simulink model "uuvSim_mfsm"  (R2017b)
settings: Solver=ode4  StartTime=0.0  StopTime=10.0  FixedStep=mdl.tStep  RelTol=1e-3
values from neighbouring files (symbols this model uses):
  trj_type = block.DialogPrm(1).Data    [trj_gen.m]    (also in trj_gen_mpc.m)
  waypoints = block.DialogPrm(2).Data    [trj_gen.m]    (also in trj_gen_mpc.m)
undefined symbols (not defined in the file or in its folder): A, ics, Kd, Ki, mdl, rov, Tinv, v_c
settings Model: Creator=e_anderlini  LastModifiedBy=e_anderlini
settings CodeAppCC: StateflowObjectComments=on

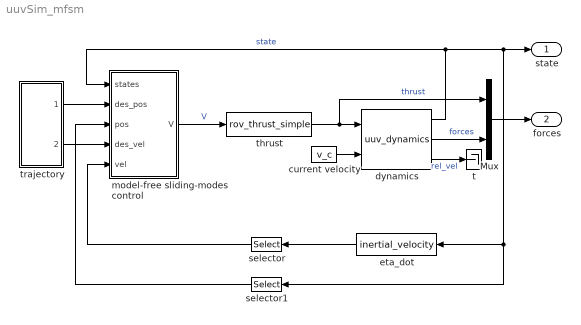
== system uuvSim_mfsm ==
  Mux : Mux  Inputs=[6,18]
  current velocity : Constant  Value=v_c
  dynamics : S-Function  FunctionName=uuv_dynamics  Parameters=rov.weight,rov.buoyancy,rov.CoG,rov.CoB,ics,rov.inv_mass',rov.M_A',rov.M_B',rov.D_l',rov.D_q'  SFunctionDeploymentMode=off  EnableBusSupport=off
  eta_dot : M-S-Function  FunctionName=inertial_velocity
  model-free sliding-modes control : Subsystem
  selector : Selector  InputPortWidth=6  IndexOptions=Index vector (dialog)  Indices=[1 2 3 6]  OutputSizes=1
  selector1 : Selector  InputPortWidth=12  IndexOptions=Index vector (dialog)  Indices=[1 2 3 6]  OutputSizes=1
  t : Terminator
  thrust : S-Function  FunctionName=rov_thrust_simple  Parameters=rov.coeffs',rov.T'  SFunctionDeploymentMode=off  EnableBusSupport=off
  trajectory : Subsystem
  state : Outport
  forces : Outport  Port=2
  wires:
  dynamics/1 -> selector1/1, eta_dot/1, state/1, model-free sliding-modes control/1(states)  "state"
  thrust/1 -> dynamics/1, Mux/1  "thrust"
  Mux/1 -> forces/1
  dynamics/2 -> Mux/2  "forces"
  model-free sliding-modes control/1(V) -> thrust/1  "V"
  dynamics/3 -> t/1  "rel_vel"
  current velocity/1 -> dynamics/2
  selector/1 -> model-free sliding-modes control/5(vel)
  trajectory/1(trj_pos) -> model-free sliding-modes control/2(des_pos)
  trajectory/2(trj_vel) -> model-free sliding-modes control/4(des_vel)
  eta_dot/1 -> selector/1
  selector1/1 -> model-free sliding-modes control/3(pos)

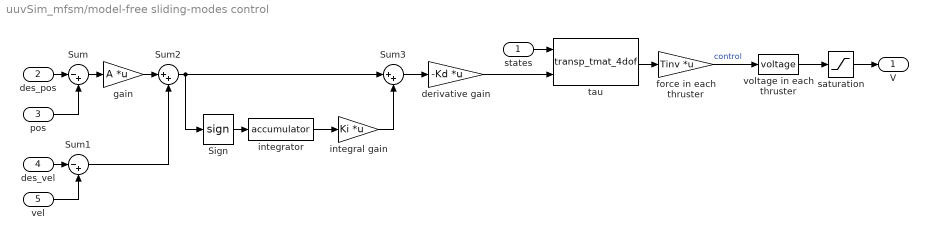
== system uuvSim_mfsm/model-free sliding-modes control ==
  states : Inport
  des_pos : Inport  Port=2
  pos : Inport  Port=3
  des_vel : Inport  Port=4
  vel : Inport  Port=5
  Sign : Signum
  Sum : Sum  Inputs=|-+
  Sum1 : Sum  Inputs=|-+
  Sum2 : Sum  Inputs=|++
  Sum3 : Sum  Inputs=|++
  derivative gain : Gain  Gain=-Kd  Multiplication=Matrix(K*u)
  force in each thruster : Gain  Gain=Tinv  Multiplication=Matrix(K*u)
  gain : Gain  Gain=A  Multiplication=Matrix(K*u)
  integral gain : Gain  Gain=Ki  Multiplication=Matrix(K*u)
  integrator : M-S-Function  FunctionName=accumulator
  saturation : Saturate  UpperLimit=5  LowerLimit=-5
  tau : S-Function  FunctionName=transp_tmat_4dof  SFunctionDeploymentMode=off  EnableBusSupport=off
  voltage in each thruster : S-Function  FunctionName=voltage  Parameters=rov.inv_coeffs'  SFunctionDeploymentMode=off  EnableBusSupport=off
  V : Outport
  wires:
  des_pos/1 -> Sum/1
  pos/1 -> Sum/2
  des_vel/1 -> Sum1/1
  vel/1 -> Sum1/2
  Sum/1 -> gain/1
  gain/1 -> Sum2/1
  Sum1/1 -> Sum2/2
  integral gain/1 -> Sum3/2
  Sum2/1 -> Sign/1, Sum3/1
  Sum3/1 -> derivative gain/1
  states/1 -> tau/1
  voltage in each thruster/1 -> saturation/1
  tau/1 -> force in each thruster/1
  derivative gain/1 -> tau/2
  force in each thruster/1 -> voltage in each thruster/1  "control"
  saturation/1 -> V/1
  Sign/1 -> integrator/1
  integrator/1 -> integral gain/1

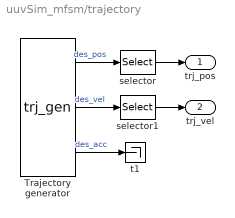
== system uuvSim_mfsm/trajectory ==
  Trajectory generator : M-S-Function  FunctionName=trj_gen  Parameters=trj_type,waypoints,mdl.tEnd,mdl.tStep
  selector : Selector  InputPortWidth=6  IndexOptions=Index vector (dialog)  Indices=[1 2 3 6]  OutputSizes=1
  selector1 : Selector  InputPortWidth=6  IndexOptions=Index vector (dialog)  Indices=[1 2 3 6]  OutputSizes=1
  t1 : Terminator
  trj_pos : Outport
  trj_vel : Outport  Port=2
  wires:
  Trajectory generator/1 -> selector/1  "des_pos"
  Trajectory generator/2 -> selector1/1  "des_vel"
  Trajectory generator/3 -> t1/1  "des_acc"
  selector/1 -> trj_pos/1
  selector1/1 -> trj_vel/1
